simulink model "sldemo_mdlref_basic"  (R2023b)
settings: Solver=FixedStepDiscrete  StartTime=0.0  StopTime=10.0  FixedStep=0.1  RelTol=1e-3
InitFcn:
  | warning('off','Simulink:Logging:DatasetRTWGenRootOutputNotSupported');
  | warning('off','Simulink:Logging:DatasetRTWGenStateNotSupported');
StartFcn:
  | warning('off','Simulink:Logging:DatasetRTWGenRootOutputNotSupported');
  | warning('off','Simulink:Logging:DatasetRTWGenStateNotSupported');
StopFcn:
  | warning('on','Simulink:Logging:DatasetRTWGenRootOutputNotSupported');
  | warning('on','Simulink:Logging:DatasetRTWGenStateNotSupported');
CloseFcn:
  | warning('on','Simulink:Logging:DatasetRTWGenRootOutputNotSupported');
  | warning('on','Simulink:Logging:DatasetRTWGenStateNotSupported');
PauseFcn:
  | warning('on','Simulink:Logging:DatasetRTWGenRootOutputNotSupported');
  | warning('on','Simulink:Logging:DatasetRTWGenStateNotSupported');
settings Model: ModifiedByFormat=The MathWorks Inc.  Creator=The MathWorks, Inc.  LastModifiedBy=The MathWorks Inc.
settings SolverCC: AlgebraicLoopSolver=TrustRegion
settings DataIOCC: LimitDataPoints=on  SaveFinalState=on  SaveState=on  SignalLoggingName=logsOut
settings OptimizationCC: DefaultParameterBehavior=Inlined  InlineInvariantSignals=on  ExpressionDepthLimit=2147483647  InitFltsAndDblsToZero=on  LifeSpan=inf
settings DebuggingCC: SaveWithParameterizedLinksMsg=none  CheckExecutionContextPreStartOutputMsg=on  MultiTaskDSMMsg=warning  MultiTaskCondExecSysMsg=none  SigSpecEnsureSampleTimeMsg=none  FcnCallInpInsideContextMsg=warning  UnconnectedInputMsg=warning  UnconnectedOutputMsg=warning  UnconnectedLineMsg=warning  AllowSymbolicDim=off  StateNameClashWarn=warning  StrictBusMsg=ErrorOnBusTreatedAsVector  SFUnexpectedBacktrackingDiag=warning  SFNoUnconditionalDefaultTransitionDiag=warning  SFExecutionAtInitializationDiag=none  ArithmeticOperatorsInVariantConditions=warning
settings HardwareCC: ProdBitPerPointer=32  ProdBitPerSizeT=32  ProdBitPerPtrDiffT=32  ProdLargestAtomicFloat=None  ProdIntDivRoundTo=Undefined  ProdEndianess=Unspecified  ProdWordSize=32  ProdHWDeviceType=32-bit Generic  TargetHWDeviceType=32-bit Generic
settings ModelReferenceCC: UpdateModelReferenceTargets=IfOutOfDate  EnableRefExpFcnMdlSchedulingChecks=on  CheckModelReferenceTargetMessage=none  PropagateSignalLabelsOutOfModel=off
settings SFSimCC: SimUseLocalCustomCode=off  CustomCodeUndefinedFunction=UseInterfaceOnly
settings RTWCC: GenerateReport=on  RTWUseLocalCustomCode=off  LaunchReport=on  DLArmComputeVersion=19.05
settings CodeAppCC: MaxIdLength=100  StateflowObjectComments=on
settings GRTTargetCC: TargetFcnLib=ansi_tfl_tmw.mat  TargetLangStandard=C89/C90 (ANSI)  CombineOutputUpdateFcns=off  GRTInterface=on
settings ConfigComp: CovMetricSettings=dw  CovSaveCumulativeToWorkspaceVar=on  CovSaveSingleToWorkspaceVar=on  CovExternalEMLEnable=off  CovSFcnEnable=off

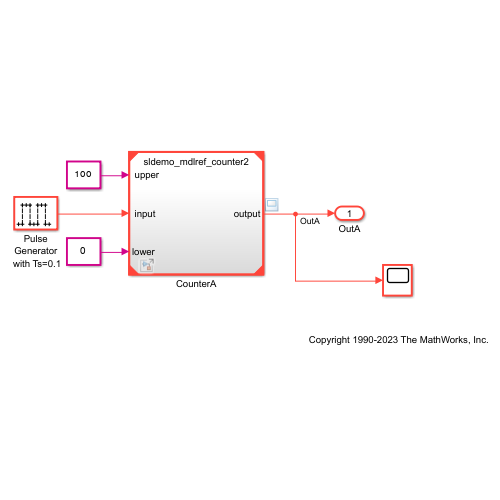
[thumbnail: Simulink's stored preview of the top-level diagram]
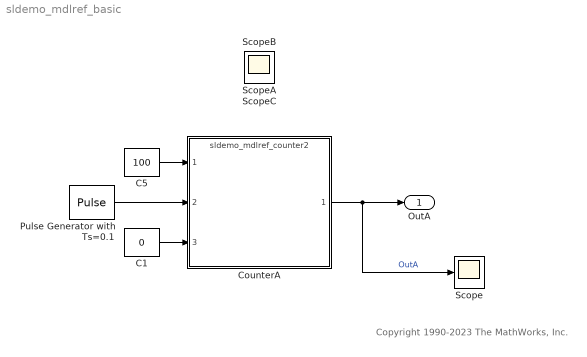
== system sldemo_mdlref_basic ==
  note: Copyright 1990-2023 The MathWorks, Inc.
  C1 : Constant  Value=0
  C5 : Constant  Value=100
  CounterA : ModelReference  ModelNameDialog=sldemo_mdlref_counter2  ModelReferenceVersion=7.10
  Pulse Generator with Ts=0.1 : DiscretePulseGenerator  SampleTime=0.1  VectorParams1D=off
  Scope : Scope
  OutA : Outport  VectorParamsAs1DForOutWhenUnconnected=off
  ScopeA : Scope
  ScopeB : Scope
  ScopeC : Scope
  wires:
  CounterA/1 -> Scope/1, OutA/1  "OutA"
  Pulse Generator with Ts=0.1/1 -> CounterA/2
  C1/1 -> CounterA/3
  C5/1 -> CounterA/1
